simulink model "mech_dpen_sticky"  (Simulink 6.0)
settings: Solver=ode45  StartTime=0.0  StopTime=20  RelTol=1e-4  AbsTol=1e-6
libraries: mblibv1 x12
settings Model: Creator=gwood  LastModifiedBy=batserve  ExtModeAutoUpdateStatusClock=off
settings DataIOCC: SignalLoggingName=sigsOut
settings OptimizationCC: BooleanDataType=off
settings DebuggingCC: AlgebraicLoopMsg=none  CheckExecutionContextPreStartOutputMsg=on  CheckExecutionContextRuntimeOutputMsg=on  SolverPrmCheckMsg=none
settings HardwareCC: TargetUnknown=on
settings SimMechanicsCC: VisOnUpdateDiagram=on  VisDuringSimulation=on

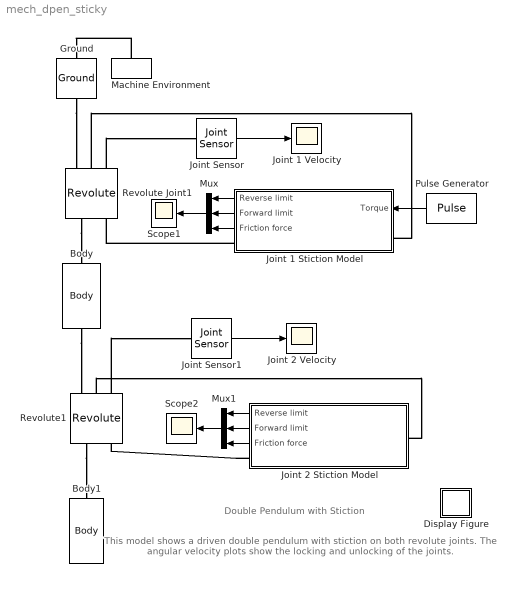
== system mech_dpen_sticky ==
  note: Double Pendulum with Stiction
  note: This model shows a driven double pendulum with stiction
      | on both revolute joints. The angular velocity plots
      | show the locking and unlocking of the joints.
  Body : mblibv1/Bodies/Body  Orientation=down  PhysicalDomain=mechanical  SubClassName=Unknown  LeftPortType=workingframe  RightPortType=workingframe  LConnTagsString=CS1  RConnTagsString=CS2  DialogClass=MechanicalBodyBlock  Mass=1  MassUnits=kg  InertiaUnits=kg*m^2  Inertia=[0.565529 0 0; 0 0.00085 0; 0 0 0.565529]  Shape=Cylinder  ShapeDims=[1 1]  ShapeUnits=m  ShapeUse=false  Density=1  DensityUnits=kg/m^3  DensityUse=false  CG=Right$CG$[0 -1 0]$WORLD$WORLD$m$[0 0 0]$Euler X-Y-Z$deg$WORLD$false  WorkingFrames=Left$CS1$[0 0 0]$WORLD$WORLD$m$[0 0 0]$Euler X-Y-Z$deg$WORLD$true#Right$CS2$[0 -2 0]$WORLD$WORLD$m$[0 0 0]$Euler X-Y-Z$deg$WORLD$true
  Body1 : mblibv1/Bodies/Body  Orientation=down  PhysicalDomain=mechanical  SubClassName=Unknown  LeftPortType=workingframe  RightPortType=workingframe  LConnTagsString=CS1  DialogClass=MechanicalBodyBlock  Mass=1  MassUnits=kg  InertiaUnits=kg*m^2  Inertia=[0.565529 0 0; 0 0.00085 0; 0 0 0.565529]  Shape=Cylinder  ShapeDims=[1 1]  ShapeUnits=m  ShapeUse=false  Density=1  DensityUnits=kg/m^3  DensityUse=false  CG=Right$CG$[0 -3 0 ]$WORLD$WORLD$m$[0 0 0]$Euler X-Y-Z$deg$WORLD$false  WorkingFrames=Left$CS1$[0 -2 0]$WORLD$WORLD$m$[0 0 0]$Euler X-Y-Z$deg$WORLD$true#Right$CS2$[0 -4 0]$WORLD$WORLD$m$[0 0 0]$Euler X-Y-Z$deg$WORLD$false
  Display Figure : Subsystem  Tag=Help  Description="Help callback for sticky double pendulum model: mech_dpen_sticky.  Opens Help browser to Type 19 marker at documentation for this tutorial model."
      settings: OpenFcn=pmhelpview([docroot '/toolbox/physmod/mech/mech.map'], 'mech_dpen_sticky_help');
      mask Type: Help callback
      mask Display: image(imread('info.bmp'))
  Ground : mblibv1/Bodies/Ground  Orientation=down  Opaque=on  LeftPortType=env  RightPortType=workingframe  PhysicalDomain=Mechanical  DialogClass=GroundBlock  CoordPosition=[0 0 0]  CoordPositionUnits=m  StateVectorMgrId=-1  MachineId=[0 0]  ShowEnvPort=on
  Joint 1 Stiction Model : Subsystem  Orientation=left
  Joint 1 Velocity : Scope
      settings: TimeRange=20  YMin=-6  YMax=8
  Joint 2 Stiction Model : Subsystem  Orientation=left
  Joint 2 Velocity : Scope
      settings: TimeRange=20  YMin=-15  YMax=10  SaveName=ScopeData3
  Joint Sensor : mblibv1/Sensors &  Actuators/Joint Sensor  Opaque=on  PhysicalDomain=Mechanical  PortType=blob  Muxed=on  Pose=off  Angle=off  AngleUnits=deg  ArcVelocity=on  ArcVelocityUnits=rad/s  ArcAcceleration=off  ArcAccelerationUnits=deg/s^2  CoordPosition=on  CoordPositionUnits=m  Velocity=off  VelocityUnits=m/s  Acceleration=off  AccelerationUnits=m/s^2  Quaternion=on  QuaternionDT=off  QuaternionDDT=off  QuaternionUnits=off  OutputVector=[ 1 ]  ActiveIO=off  Width=1  DialogClass=MechanicalSensorBlock  Primitive=R1  Force=off  ForceUnits=N  Torque=off  TorqueUnits=N-m  ReferenceFrame=Absolute (INERTIAL)  ReactionSensedSide=Base  ReactionReferenceFrame=Absolute (World)  ReactionForce=off  ReactionForceUnits=N  ReactionMoment=off  ReactionMomentUnits=N-m
  Joint Sensor1 : mblibv1/Sensors &  Actuators/Joint Sensor  Opaque=on  PhysicalDomain=Mechanical  PortType=blob  Muxed=on  Pose=off  Angle=off  AngleUnits=deg  ArcVelocity=on  ArcVelocityUnits=rad/s  ArcAcceleration=off  ArcAccelerationUnits=deg/s^2  CoordPosition=on  CoordPositionUnits=m  Velocity=off  VelocityUnits=m/s  Acceleration=off  AccelerationUnits=m/s^2  Quaternion=on  QuaternionDT=off  QuaternionDDT=off  QuaternionUnits=off  OutputVector=[ 1 ]  ActiveIO=off  Width=1  DialogClass=MechanicalSensorBlock  Primitive=R1  Force=off  ForceUnits=N  Torque=off  TorqueUnits=N-m  ReferenceFrame=Absolute (INERTIAL)  ReactionSensedSide=Base  ReactionReferenceFrame=Absolute (World)  ReactionForce=off  ReactionForceUnits=N  ReactionMoment=off  ReactionMomentUnits=N-m
  Machine Environment : mblibv1/Bodies/Machine Environment  Tag=Factory ground  Orientation=up  DialogController=MECH.DialogSource  Opaque=on  PortType=env  PhysicalDomain=Mechanical  DialogTemplateClass=MECH.MachineEnvironment  SyncWhenCopied=off  Gravity=[0 -9.81 0]  GravityUnits=m/s^2  GravityAsSignal=off  Dimensionality=3D Only  AnalysisType=Forward dynamics  LinearAssemblyTolerance=1e-3  LinearAssemblyToleranceUnits=m  AngularAssemblyTolerance=1e-3  AngularAssemblyToleranceUnits=rad  ConstraintSolverType=Machine precision  ConstraintRelTolerance=1e-4  ConstraintAbsTolerance=1e-4  UseRobustSingularityHandling=off  StatePerturbationType=Fixed  PerturbationSize=1e-5  VisualizeMachine=on
  Mux : Mux  Orientation=left  Inputs=3
  Mux1 : Mux  Orientation=left  Inputs=3
  Pulse Generator : DiscretePulseGenerator  Orientation=left  PulseType=Time based  Amplitude=50  Period=15  PulseWidth=5
  Revolute Joint1 : mblibv1/Joints/Revolute  Orientation=down  PhysicalDomain=mechanical  SubClassName=Unknown  LeftPortType=blob  RightPortType=blob  LConnTagsString=__newl0|SA1|SA2  RConnTagsString=__newr0|SA1  NumSAPorts=3  CutJoint=off  MarkAsCut=off  Primitives=revolute  PrimitiveProps=R1$WORLD$[0 0 1 ]$revolute  DialogClass=JointBlock
  Revolute1 : mblibv1/Joints/Revolute  Orientation=down  PhysicalDomain=mechanical  SubClassName=Unknown  LeftPortType=blob  RightPortType=blob  LConnTagsString=__newl0|SA1|SA2  RConnTagsString=__newr0|SA1  NumSAPorts=3  CutJoint=off  MarkAsCut=off  Primitives=revolute  PrimitiveProps=R1$WORLD$[0 0 1 ]$revolute  DialogClass=JointBlock
  Scope1 : Scope
      settings: TimeRange=10  YMin=-80  YMax=80
  Scope2 : Scope
      settings: TimeRange=10  YMin=-15  YMax=15  SaveName=ScopeData2
  wires:
  Joint 1 Stiction Model/1(Reverse limit) -> Mux/1
  Joint 1 Stiction Model/2(Forward limit) -> Mux/2
  Joint 1 Stiction Model/3(Friction force) -> Mux/3
  Mux/1 -> Scope1/1
  Joint Sensor/1 -> Joint 1 Velocity/1
  Mux1/1 -> Scope2/1
  Joint 2 Stiction Model/1(Reverse limit) -> Mux1/1
  Joint 2 Stiction Model/2(Forward limit) -> Mux1/2
  Joint 2 Stiction Model/3(Friction force) -> Mux1/3
  Joint Sensor1/1 -> Joint 2 Velocity/1
  Pulse Generator/1 -> Joint 1 Stiction Model/1(Torque)
  connections:
  Ground/RConn1 -- Revolute Joint1/LConn1
  Revolute Joint1/RConn1 -- Body/LConn1
  Body/RConn1 -- Revolute1/LConn1
  Revolute1/RConn1 -- Body1/LConn1
  Revolute Joint1/LConn3 -- Joint Sensor/LConn1
  Revolute1/LConn3 -- Joint Sensor1/LConn1
  Joint 1 Stiction Model/RConn1 -- Revolute Joint1/RConn2
  Revolute Joint1/LConn2 -- Joint 1 Stiction Model/LConn1
  Revolute1/LConn2 -- Joint 2 Stiction Model/LConn1
  Joint 2 Stiction Model/RConn1 -- Revolute1/RConn2
  Machine Environment/RConn1 -- Ground/LConn1

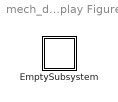
== system mech_dpen_sticky/Display Figure ==
  EmptySubsystem : Subsystem

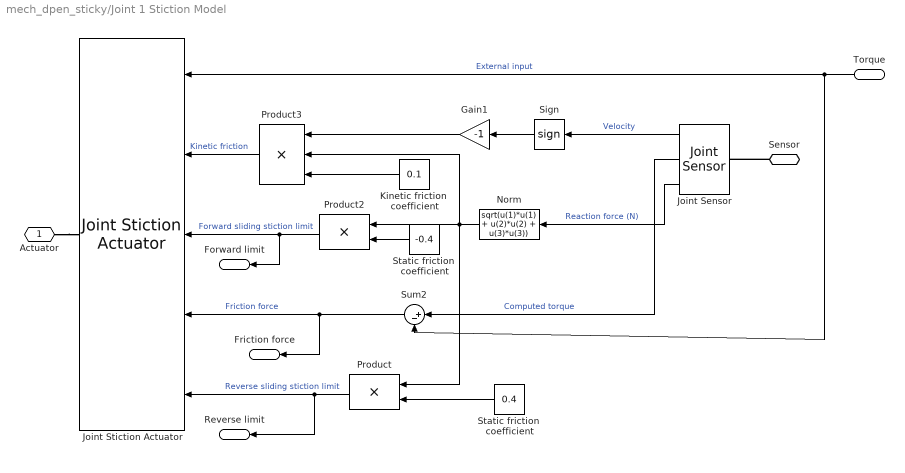
== system mech_dpen_sticky/Joint 1 Stiction Model ==
  Torque : Inport  Orientation=left  Port=1  LatchInput=off
  Gain1 : Gain  Orientation=left  Gain=-1  SaturateOnIntegerOverflow=on
  Joint Sensor : mblibv1/Sensors &  Actuators/Joint Sensor  Orientation=left  Opaque=on  PhysicalDomain=Mechanical  PortType=blob  Muxed=off  Pose=off  Angle=off  AngleUnits=deg  ArcVelocity=on  ArcVelocityUnits=deg/s  ArcAcceleration=off  ArcAccelerationUnits=deg/s^2  CoordPosition=on  CoordPositionUnits=m  Velocity=off  VelocityUnits=m/s  Acceleration=off  AccelerationUnits=m/s^2  Quaternion=on  QuaternionDT=off  QuaternionDDT=off  QuaternionUnits=off  OutputVector=[ 1 1 3 ]  ActiveIO=off  Width=1  DialogClass=MechanicalSensorBlock  Primitive=R1  Force=off  ForceUnits=N  Torque=on  TorqueUnits=N-m  ReferenceFrame=Absolute (INERTIAL)  ReactionSensedSide=Base  ReactionReferenceFrame=Absolute (World)  ReactionForce=on  ReactionForceUnits=N  ReactionMoment=off  ReactionMomentUnits=N-m
  Joint Stiction Actuator : mblibv1/Sensors &  Actuators/Joint Stiction Actuator  Orientation=left  Opaque=on  PhysicalDomain=Mechanical  PortType=blob  ActuationStyle=Force  AngleUnits=deg  ArcVelocityUnits=deg/s  ArcAccelerationUnits=deg/s^2  CoordPositionUnits=m  VelocityUnits=m/s  AccelerationUnits=m/s^2  ForceUnits=N  TorqueUnits=N-m  ActiveIO=off  Width=1  DialogClass=EventActuatorBlock  Primitive=R1  FrictionalForceUnits=N-m  ExternalForceUnits=N-m  FrictionalTorqueUnits=N-m  ExternalTorqueUnits=N-m  LockingTolerance=1e-3
  Kinetic friction  coefficient : Constant  Orientation=left  Value=0.1
  Norm : Fcn  Orientation=left  Expr=sqrt(u(1)*u(1) + u(2)*u(2) + u(3)*u(3))
  Product : Product  Orientation=left  SaturateOnIntegerOverflow=on  InputSameDT=on
  Product2 : Product  Orientation=left  SaturateOnIntegerOverflow=on  InputSameDT=on
  Product3 : Product  Orientation=left  Inputs=3  SaturateOnIntegerOverflow=on  InputSameDT=on
  Sign : Signum  Orientation=left  ZeroCross=off
  Static friction  coefficient : Constant  Orientation=left  Value=0.4
  "Static friction  coefficient " : Constant  Orientation=left  Value=-0.4
  Sum2 : Sum  Orientation=left  Inputs=|+-  SaturateOnIntegerOverflow=on  InputSameDT=on
  Actuator : PMIOPort  Port=1  Side=Right
  Sensor : PMIOPort  Orientation=left  Port=2  Side=Left
  Reverse limit : Outport  Orientation=left
  Forward limit : Outport  Orientation=left  Port=2
  Friction force : Outport  Orientation=left  Port=3
  wires:
  Joint Sensor/1 -> Sign/1  "Velocity"
  Sign/1 -> Gain1/1
  Joint Sensor/3 -> Norm/1  "Reaction force (N)"
  Product/1 -> Reverse limit/1, Joint Stiction Actuator/5  "Reverse sliding stiction limit"
  Product2/1 -> Forward limit/1, Joint Stiction Actuator/3  "Forward sliding stiction limit"
  Norm/1 -> Product3/2, Product2/1, Product/1
  Gain1/1 -> Product3/1
  Kinetic friction  coefficient/1 -> Product3/3
  Product3/1 -> Joint Stiction Actuator/2  "Kinetic friction"
  Static friction  coefficient/1 -> Product/2
  Joint Sensor/2 -> Sum2/1  "Computed torque"
  Sum2/1 -> Joint Stiction Actuator/4, Friction force/1  "Friction force"
  Torque/1 -> Joint Stiction Actuator/1, Sum2/2  "External input"
  "Static friction  coefficient "/1 -> Product2/2
  connections:
  Actuator/RConn1 -- Joint Stiction Actuator/RConn1
  Sensor/RConn1 -- Joint Sensor/LConn1

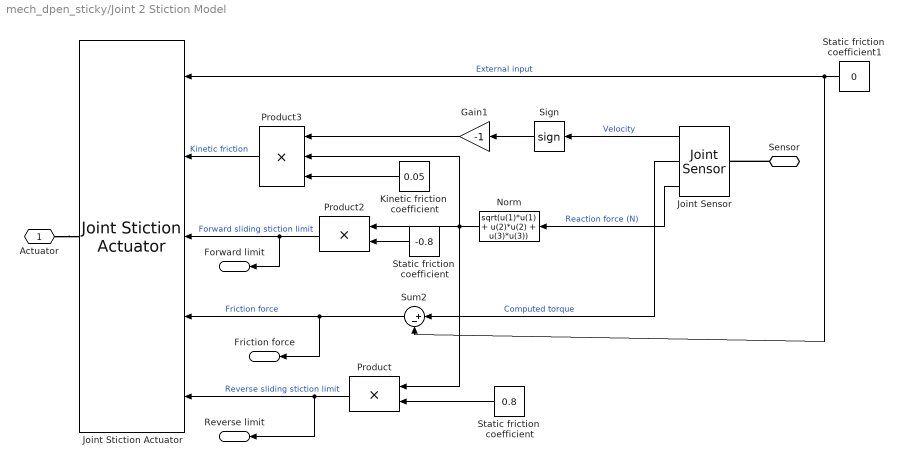
== system mech_dpen_sticky/Joint 2 Stiction Model ==
  Gain1 : Gain  Orientation=left  Gain=-1  SaturateOnIntegerOverflow=on
  Joint Sensor : mblibv1/Sensors &  Actuators/Joint Sensor  Orientation=left  Opaque=on  PhysicalDomain=Mechanical  PortType=blob  Muxed=off  Pose=off  Angle=off  AngleUnits=deg  ArcVelocity=on  ArcVelocityUnits=deg/s  ArcAcceleration=off  ArcAccelerationUnits=deg/s^2  CoordPosition=on  CoordPositionUnits=m  Velocity=off  VelocityUnits=m/s  Acceleration=off  AccelerationUnits=m/s^2  Quaternion=on  QuaternionDT=off  QuaternionDDT=off  QuaternionUnits=off  OutputVector=[ 1 1 3 ]  ActiveIO=off  Width=1  DialogClass=MechanicalSensorBlock  Primitive=R1  Force=off  ForceUnits=N  Torque=on  TorqueUnits=N-m  ReferenceFrame=Absolute (INERTIAL)  ReactionSensedSide=Base  ReactionReferenceFrame=Absolute (World)  ReactionForce=on  ReactionForceUnits=N  ReactionMoment=off  ReactionMomentUnits=N-m
  Joint Stiction Actuator : mblibv1/Sensors &  Actuators/Joint Stiction Actuator  Orientation=left  Opaque=on  PhysicalDomain=Mechanical  PortType=blob  ActuationStyle=Force  AngleUnits=deg  ArcVelocityUnits=deg/s  ArcAccelerationUnits=deg/s^2  CoordPositionUnits=m  VelocityUnits=m/s  AccelerationUnits=m/s^2  ForceUnits=N  TorqueUnits=N-m  ActiveIO=off  Width=1  DialogClass=EventActuatorBlock  Primitive=R1  FrictionalForceUnits=N-m  ExternalForceUnits=N-m  FrictionalTorqueUnits=N-m  ExternalTorqueUnits=N-m  LockingTolerance=1e-3
  Kinetic friction  coefficient : Constant  Orientation=left  Value=0.05
  Norm : Fcn  Orientation=left  Expr=sqrt(u(1)*u(1) + u(2)*u(2) + u(3)*u(3))
  Product : Product  Orientation=left  SaturateOnIntegerOverflow=on  InputSameDT=on
  Product2 : Product  Orientation=left  SaturateOnIntegerOverflow=on  InputSameDT=on
  Product3 : Product  Orientation=left  Inputs=3  SaturateOnIntegerOverflow=on  InputSameDT=on
  Sign : Signum  Orientation=left  ZeroCross=off
  Static friction  coefficient : Constant  Orientation=left  Value=0.8
  "Static friction  coefficient " : Constant  Orientation=left  Value=-0.8
  Static friction  coefficient1 : Constant  Orientation=left  Value=0
  Sum2 : Sum  Orientation=left  Inputs=|+-  SaturateOnIntegerOverflow=on  InputSameDT=on
  Actuator : PMIOPort  Port=1  Side=Right
  Sensor : PMIOPort  Orientation=left  Port=2  Side=Left
  Reverse limit : Outport  Orientation=left
  Forward limit : Outport  Orientation=left  Port=2
  Friction force : Outport  Orientation=left  Port=3
  wires:
  "Static friction  coefficient "/1 -> Product2/2
  Static friction  coefficient1/1 -> Sum2/2, Joint Stiction Actuator/1  "External input"
  Sum2/1 -> Friction force/1, Joint Stiction Actuator/4  "Friction force"
  Joint Sensor/2 -> Sum2/1  "Computed torque"
  Static friction  coefficient/1 -> Product/2
  Product3/1 -> Joint Stiction Actuator/2  "Kinetic friction"
  Kinetic friction  coefficient/1 -> Product3/3
  Gain1/1 -> Product3/1
  Norm/1 -> Product/1, Product2/1, Product3/2
  Product2/1 -> Joint Stiction Actuator/3, Forward limit/1  "Forward sliding stiction limit"
  Product/1 -> Joint Stiction Actuator/5, Reverse limit/1  "Reverse sliding stiction limit"
  Joint Sensor/3 -> Norm/1  "Reaction force (N)"
  Sign/1 -> Gain1/1
  Joint Sensor/1 -> Sign/1  "Velocity"
  connections:
  Sensor/RConn1 -- Joint Sensor/LConn1
  Actuator/RConn1 -- Joint Stiction Actuator/RConn1

== system mech_dpen_sticky/Display Figure/EmptySubsystem ==
